simulink subsystem "ConvertTheta"  (R2024a)
settings: Solver=VariableStepAuto  StartTime=0.0  StopTime=10.0  RelTol=1e-3
libraries: simulink x2
settings Model: Creator=44779  LastModifiedBy=44779

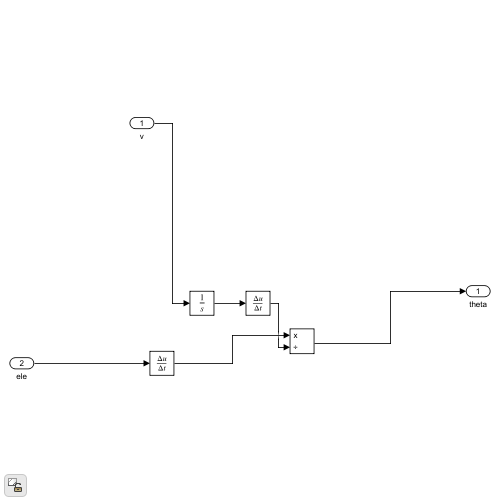
[thumbnail: Simulink's stored preview of the top-level diagram]
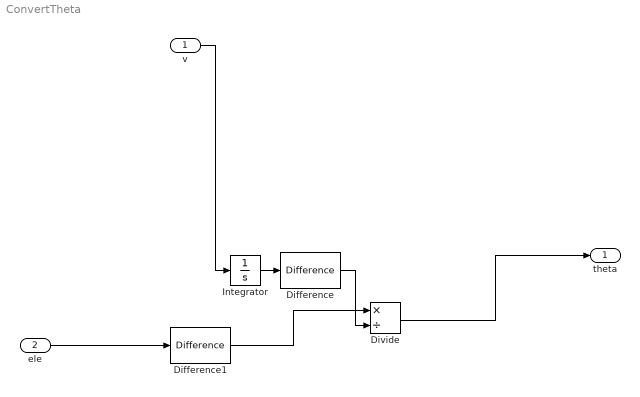
== system ConvertTheta ==
  v : Inport
  ele : Inport  Port=2
  Difference : simulink/Discrete/Difference  ICPrevInput=0.0  OutMin=[]  OutMax=[]  OutDataType=fixdt(1, 16)  OutScaling=2^-10  DoSatur=off
  Difference1 : simulink/Discrete/Difference  ICPrevInput=0.0  OutMin=[]  OutMax=[]  OutDataType=fixdt(1, 16)  OutScaling=2^-10  DoSatur=off
  Divide : Product  Inputs=*/
  Integrator : Integrator
  theta : Outport
  wires:
  Difference/1 -> Divide/2
  Integrator/1 -> Difference/1
  Difference1/1 -> Divide/1
  Divide/1 -> theta/1
  v/1 -> Integrator/1
  ele/1 -> Difference1/1
